simulink model "chap7_15"  (Simulink 3.00)
settings: Solver=ode4  StartTime=0.0  StopTime=200  RelTol=1e-3
values from neighbouring files (symbols this model uses):
  alfa = 1.0    (= 1)    [chap7_14.m]    (also in chap7_15f.m)
  kd = 0.20    (= 0.2)    [chap7_10.m]    (also in chap7_14.m = 0.01; chap7_15f.m = 1; chap7_2.m = 15; chap7_3f.m = 1.9688)
  ki = 0.80    (= 0.8)    [chap7_10.m]    (also in chap7_14.m = 0.01; chap7_15f.m = 10; chap7_2.m = 0; chap7_3f.m = 0.0504)
  kp = 8.0    (= 8)    [chap7_10.m]    (also in chap7_14.m = 0.1; chap7_15f.m = 50; chap7_2.m = 50; chap7_3f.m = 0.63)
  umax = 10    [chap7_14.m]    (also in chap7_15f.m; chap7_15m.m)
  umin = 0    [chap7_14.m]    (also in chap7_15f.m; chap7_15m.m)
undefined symbols (not defined in the file or in its folder): chap7_15m
settings Model: SaveTime=off  SaveOutput=off  Decimation=100

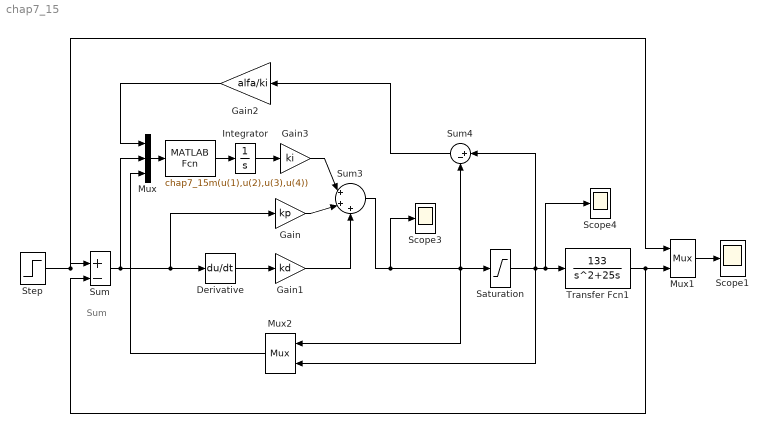
== system chap7_15 ==
  note: Sum
  "    " : MATLABFcn  MATLABFcn=chap7_15m(u(1),u(2),u(3),u(4))  OutputWidth=1  OutputSignalType=auto
  Derivative : Derivative
  Gain : Gain  Gain=kp  SaturateOnIntegerOverflow=on
  Gain1 : Gain  Gain=kd  SaturateOnIntegerOverflow=on
  Gain2 : Gain  Orientation=left  Gain=alfa/ki  SaturateOnIntegerOverflow=on
  Gain3 : Gain  Gain=ki  SaturateOnIntegerOverflow=on
  Integrator : Integrator  ExternalReset=none  InitialConditionSource=internal  InitialCondition=0  LimitOutput=off  UpperSaturationLimit=inf  LowerSaturationLimit=-inf  ShowSaturationPort=off  ShowStatePort=off  AbsoluteTolerance=auto
  Mux : Mux  Inputs=3
  Mux1 : Mux  Inputs=2
      settings: DisplayOption=none
  Mux2 : Mux  Orientation=left  Inputs=2
      settings: DisplayOption=none
  Saturation : Saturate  UpperLimit=umax  LowerLimit=umin
  Scope1 : Scope
      settings: TimeRange=0.2  YMin=1470  YMax=1500  SaveToWorkspace=off  SaveName=ScopeData  MaxRows=500000  Decimation=0.001  SampleInput=on  SampleTime=0.001
  Scope3 : Scope
      settings: TimeRange=0.2  YMin=-0.051  YMax=-0.041  SaveToWorkspace=off  SaveName=ScopeData  MaxRows=500000  Decimation=0.001  SampleInput=on  SampleTime=0.001
  Scope4 : Scope
      settings: TimeRange=0.2  YMin=-0.051  YMax=-0.041  SaveToWorkspace=off  SaveName=ScopeData  MaxRows=500000  Decimation=0.001  SampleInput=on  SampleTime=0.001
  Step : Step  Time=0  Before=0  After=1500  SampleTime=0
  Sum : Sum  Inputs=|+-  SaturateOnIntegerOverflow=on
  Sum3 : Sum  Inputs=|+++  SaturateOnIntegerOverflow=on
  Sum4 : Sum  Orientation=left  Inputs=|+-  SaturateOnIntegerOverflow=on
  Transfer Fcn1 : TransferFcn  Numerator=[133]  Denominator=[1 25 0]
  wires:
  Mux1/1 -> Scope1/1
  Transfer Fcn1/1 -> Mux1/2, Sum/2
  Derivative/1 -> Gain1/1
  Sum3/1 -> Scope3/1, Saturation/1, Sum4/2, Mux2/1
  Saturation/1 -> Transfer Fcn1/1, Scope4/1, Sum4/1, Mux2/2
  Gain1/1 -> Sum3/3
  Gain/1 -> Sum3/2
  Step/1 -> Sum/1, Mux1/1
  Gain3/1 -> Sum3/1
  Integrator/1 -> Gain3/1
  Sum4/1 -> Gain2/1
  "    "/1 -> Integrator/1
  Mux/1 -> "    "/1
  Gain2/1 -> Mux/1
  Sum/1 -> Gain/1, Derivative/1, Mux/2
  Mux2/1 -> Mux/3
